simulink model "lag_submodule"  (R2018b)
settings: Solver=VariableStepAuto  StartTime=0.0  StopTime=10.0  RelTol=1e-3
settings Model: Creator=jh2044  LastModifiedBy=jh2044

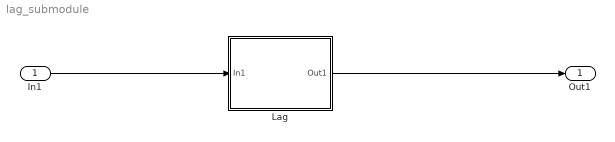
== system lag_submodule ==
  In1 : Inport
  Lag : Subsystem
  Out1 : Outport
  wires:
  In1/1 -> Lag/1(In1)
  Lag/1(Out1) -> Out1/1

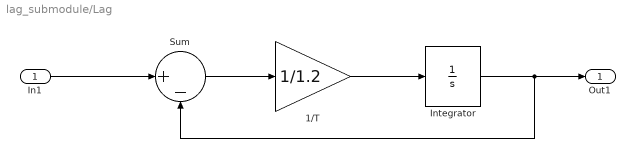
== system lag_submodule/Lag ==
  In1 : Inport
  1/T : Gain  Gain=1/1.2
  Integrator : Integrator
  Sum : Sum  Inputs=|+-
  Out1 : Outport
  wires:
  1/T/1 -> Integrator/1
  Integrator/1 -> Out1/1, Sum/2
  In1/1 -> Sum/1
  Sum/1 -> 1/T/1
